simulink model "controlsystem"  (R2015a)
settings: Solver=ode45  StartTime=0.0  StopTime=20  RelTol=1e-3
settings Model: Creator=tvincent  LastModifiedBy=tvincent
settings DebuggingCC: UnderspecifiedInitializationDetection=Classic  MergeDetectMultiDrivingBlocksExec=none  SolverPrmCheckMsg=warning

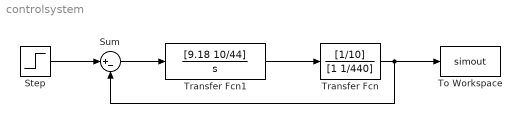
== system controlsystem ==
  Step : Step  Time=0  SampleTime=0
  Sum : Sum  Inputs=|+-
  To Workspace : ToWorkspace  VariableName=simout  SaveFormat=Structure With Time  SampleTime=-1
  Transfer Fcn : TransferFcn  Numerator=[1/10]  Denominator=[1 1/440]
  Transfer Fcn1 : TransferFcn  Numerator=[9.18 10/44]  Denominator=[1 0]
  wires:
  Transfer Fcn1/1 -> Transfer Fcn/1
  Sum/1 -> Transfer Fcn1/1
  Transfer Fcn/1 -> To Workspace/1, Sum/2
  Step/1 -> Sum/1
